simulink model "Data_Center_Module_Tier_1_No_Switching"  (R2024b)
settings: Solver=VariableStepAuto  StartTime=0.0  StopTime=60  RelTol=1e-3
undefined symbols (not defined in the file or in its folder): D1, Delta
libraries: spsThreePhaseSeriesRLCBranchLib x8, spsThreePhaseSeriesRLCLoadLib x7, spsThreePhaseProgrammableVoltageSourceLib x3, spsGroundLib x3, spsThreePhaseBreakerLib x3, spsThreePhaseTransformerTwoWindingsLib x2, spsPower3phInstantaneousLib x1, spsThreePhaseVIMeasurementLib x1, sps_lib x1
settings Model: Creator=Kapla  LastModifiedBy=Kapla

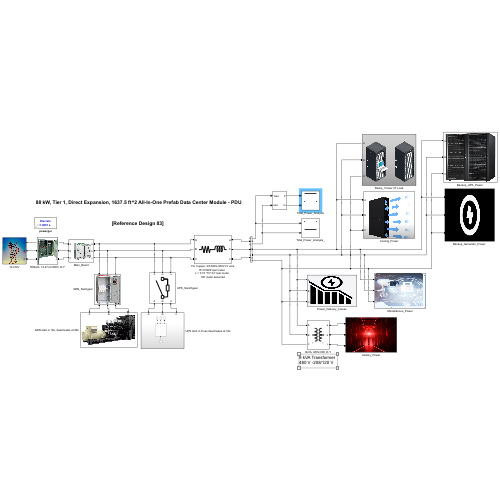
[thumbnail: Simulink's stored preview of the top-level diagram]
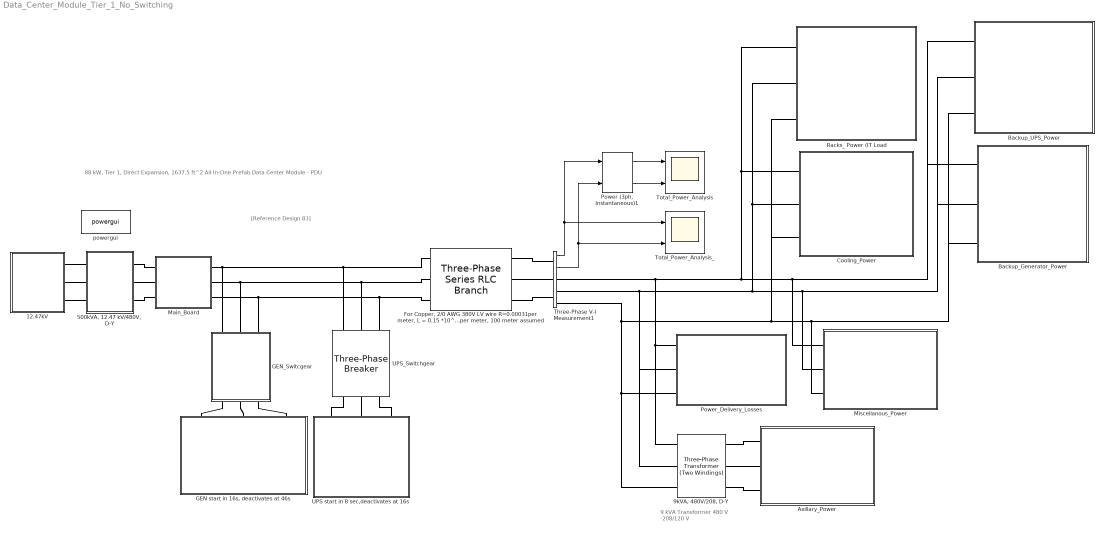
== system Data_Center_Module_Tier_1_No_Switching ==
  note: 9 kVA Transformer
      | 480 V -208/120 V
  note: [Reference Design 83]
  note: 88 kW, Tier 1, Direct Expansion, 1637.5 ft^2 All-In-One Prefab Data Center Module - PDU
  12.47kV : Subsystem
      mask Display: image('Power_Grid_.png');
  "500kVA, 12.47 kV/480V, D-Y" : Subsystem
      mask Display: image('Data_Center_Transformer_Tier_1.png');
  "9kVA, 480V/208, D-Y" : spsThreePhaseTransformerTwoWindingsLib/Three-Phase Transformer (Two Windings)  Winding1Connection=Y  Winding2Connection=Y  CoreType=Three single-phase transformers  SetSaturation=off  Hysteresis=off  DataFile='hysteresis'  SetInitialFlux=off  Measurements=None  UNITS=pu  NominalPower=[9e3 , 60 ]  Winding1=[ 480 , 0.002 , 0.08 ]  Winding2=[208 , 0.002 , 0.08 ]  Rm=500  Lm=500  L0=0.5  Saturation=[ 0,0 ; 0.0024,1.2 ; 1.0,1.52 ]  InitialFluxes=[ 0.8 , -0.8 , 0.7 ]  BreakLoop=off  DiscreteSolver=Trapezoidal iterative  DataType=off  TransfoNumber=1
  Axiliary_Power : Subsystem
      mask Display: image('Lighting_monitoring.png');
  "Backup_Generator_Power " : Subsystem
      mask Display: image('back up_generator_power.png');
  "Backup_UPS_Power " : Subsystem
      mask Display: image('UPS.png');
  Cooling_Power : Subsystem
      mask Display: image('Coolin.png');
  "For Copper, 2/0 AWG 380V LV wire R=0.00031per meter, L = 0.15 *10^-6 H per meter, 100 meter assumed " : spsThreePhaseSeriesRLCBranchLib/Three-Phase Series RLC Branch  LConnTagsString=A|B|C  RConnTagsString=A|B|C  BranchType=RL  Resistance=0.00031*100  Inductance=0.15e-6*100  Capacitance=[]  Measurements=None
  "GEN start in 16s, deactivates at 46s" : Subsystem
      mask Display: image('Back_up_Generator.png');
  GEN_Switcgear : Subsystem
      mask Display: image('GEN_Switch_gear_500kW.png');
  Main_Board : Subsystem
      mask Display: image('Main_Switch_Gear_Board.png');
  Miscellanous_Power : Subsystem
      mask Display: image('Data_Center_Security.png');
  "Power (3ph, Instantaneous)1" : spsPower3phInstantaneousLib/Power (3ph, Instantaneous)
  Power_Delivery_Losses : Subsystem
      mask Display: image('Power_Delivery_losses.png');
  Racks_ Power (IT Load : Subsystem
      mask Display: image('racks_server.png');
  Three-Phase V-I Measurement1 : spsThreePhaseVIMeasurementLib/Three-Phase V-I Measurement  VoltageMeasurement=phase-to-ground  SetLabelV=off  LabelV=V1  Vpu=off  VpuLL=off  CurrentMeasurement=yes  SetLabelI=off  LabelI=I1  Ipu=off  Pbase=100e6  Vbase=500e3  OutputType=Magnitude  PhasorSimulation=off  PSBequivalent=0
  Total_Power_Analysis : Scope  NumInputPorts=2
  Total_Power_Analysis_ : Scope  NumInputPorts=2
  UPS start in 8 sec,deactivates at 16s : Subsystem
  UPS_Switchgear : spsThreePhaseBreakerLib/Three-Phase Breaker  InitialState=open  SwitchA=on  SwitchB=on  SwitchC=on  SwitchTimes=[8 16]  External=off  BreakerResistance=0.01  SnubberResistance=1e6  SnubberCapacitance=inf  Measurements=None
  powergui : sps_lib/powergui  Priority=1  SimulationMode=Discrete  SampleTime=100e-6  frequency=60  Iterations=50  frequencyindice=60  Pbase=100e6  ErrMax=1e-4  UnitsV=kV  UnitsW=MW  buscounter=0  FunctionMessages=off  echomessages=off  EnableUseOfTLC=off  CurrentSourceSwitches=off  DisableSnubberDevices=off  DisableRonSwitches=off  DisableVfSwitches=off  DisplayEquations=off  AutomaticDiscreteSolvers=off  SolverType=Tustin/Backward Euler (TBE)  Interpol=off  ExternalGateDelay=off  methode=off  Ts=100  x0status=blocks  SPID=on  SwTol=0  HookPort=off  NonlinearTolerance=1e-4  nMaxIteration=100  ContinueOnMaxIteration=off  RestoreLinks=warning  ResistiveCurrentMeasurement=off  Frange=[0:2:500]  Ylog=off  Xlog=on  ShowGrid=off  save=off  variable=ZData  structure=0  ZoomFFT=off  StartTime=0.0  cycles=1  DisplayStyle=1  fundamental=60  FreqAxis=off  MaxFrequency=1000  frequencyindicesteady=1  RmsSteady=1  display=off
  wires:
  "Power (3ph, Instantaneous)1"/2 -> Total_Power_Analysis/2
  Three-Phase V-I Measurement1/1 -> "Power (3ph, Instantaneous)1"/1, Total_Power_Analysis_/1
  "Power (3ph, Instantaneous)1"/1 -> Total_Power_Analysis/1
  Three-Phase V-I Measurement1/2 -> "Power (3ph, Instantaneous)1"/2, Total_Power_Analysis_/2
  connections:
  Power_Delivery_Losses/LConn1 -- "9kVA, 480V/208, D-Y"/LConn1 -- "Backup_UPS_Power "/LConn1 -- "Backup_Generator_Power "/LConn1 -- Miscellanous_Power/LConn1 -- Racks_ Power (IT Load/LConn1 -- Cooling_Power/LConn1 -- Three-Phase V-I Measurement1/RConn1
  "For Copper, 2/0 AWG 380V LV wire R=0.00031per meter, L = 0.15 *10^-6 H per meter, 100 meter assumed "/RConn1 -- Three-Phase V-I Measurement1/LConn1
  "For Copper, 2/0 AWG 380V LV wire R=0.00031per meter, L = 0.15 *10^-6 H per meter, 100 meter assumed "/RConn3 -- Three-Phase V-I Measurement1/LConn3
  "9kVA, 480V/208, D-Y"/LConn2 -- Power_Delivery_Losses/LConn2 -- Three-Phase V-I Measurement1/RConn2 -- "Backup_UPS_Power "/LConn2 -- "Backup_Generator_Power "/LConn2 -- Miscellanous_Power/LConn2 -- Racks_ Power (IT Load/LConn2 -- Cooling_Power/LConn2
  Power_Delivery_Losses/LConn3 -- "9kVA, 480V/208, D-Y"/LConn3 -- "Backup_UPS_Power "/LConn3 -- "Backup_Generator_Power "/LConn3 -- Miscellanous_Power/LConn3 -- Racks_ Power (IT Load/LConn3 -- Cooling_Power/LConn3 -- Three-Phase V-I Measurement1/RConn3
  "For Copper, 2/0 AWG 380V LV wire R=0.00031per meter, L = 0.15 *10^-6 H per meter, 100 meter assumed "/RConn2 -- Three-Phase V-I Measurement1/LConn2
  Axiliary_Power/LConn1 -- "9kVA, 480V/208, D-Y"/RConn1
  Axiliary_Power/LConn3 -- "9kVA, 480V/208, D-Y"/RConn3
  Axiliary_Power/LConn2 -- "9kVA, 480V/208, D-Y"/RConn2
  UPS_Switchgear/LConn1 -- UPS start in 8 sec,deactivates at 16s/RConn1
  UPS_Switchgear/LConn2 -- UPS start in 8 sec,deactivates at 16s/RConn2
  UPS_Switchgear/LConn3 -- UPS start in 8 sec,deactivates at 16s/RConn3
  12.47kV/RConn1 -- "500kVA, 12.47 kV/480V, D-Y"/LConn1
  12.47kV/RConn2 -- "500kVA, 12.47 kV/480V, D-Y"/LConn2
  12.47kV/RConn3 -- "500kVA, 12.47 kV/480V, D-Y"/LConn3
  GEN_Switcgear/LConn1 -- "GEN start in 16s, deactivates at 46s"/RConn1
  GEN_Switcgear/LConn2 -- "GEN start in 16s, deactivates at 46s"/RConn2
  GEN_Switcgear/LConn3 -- "GEN start in 16s, deactivates at 46s"/RConn3
  "For Copper, 2/0 AWG 380V LV wire R=0.00031per meter, L = 0.15 *10^-6 H per meter, 100 meter assumed "/LConn3 -- Main_Board/RConn3 -- GEN_Switcgear/RConn3 -- UPS_Switchgear/RConn3
  GEN_Switcgear/RConn2 -- Main_Board/RConn2 -- UPS_Switchgear/RConn2 -- "For Copper, 2/0 AWG 380V LV wire R=0.00031per meter, L = 0.15 *10^-6 H per meter, 100 meter assumed "/LConn2
  GEN_Switcgear/RConn1 -- Main_Board/RConn1 -- UPS_Switchgear/RConn1 -- "For Copper, 2/0 AWG 380V LV wire R=0.00031per meter, L = 0.15 *10^-6 H per meter, 100 meter assumed "/LConn1
  Main_Board/LConn1 -- "500kVA, 12.47 kV/480V, D-Y"/RConn1
  "500kVA, 12.47 kV/480V, D-Y"/RConn2 -- Main_Board/LConn2
  Main_Board/LConn3 -- "500kVA, 12.47 kV/480V, D-Y"/RConn3

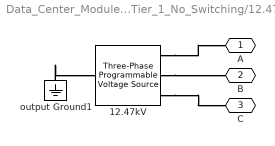
== system Data_Center_Module_Tier_1_No_Switching/12.47kV ==
  12.47kV : spsThreePhaseProgrammableVoltageSourceLib/Three-Phase Programmable Voltage Source  PositiveSequence="[12.4e3 0  60]"  VariationEntity=None  VariationType=Step  VariationTypeAlt=Step  VariationStep=-0.5  VariationRate=10  VariationMagnitude=0.5  VariationFrequency=1  VariationTiming=[0.2 1.2]  VariationPhaseA=off  Amplitudes=[1 0.8 1.2 1.0]  TimeValues=[0 0.1 0.15 0.2]  HarmonicGeneration=off  HarmonicA=[3 0.2 -25 0]  HarmonicB="[2 0.15  35 2]"  Timing="[0.05  3]"  BusType=swing  Pref=0  Qref=0  Qmin=-inf  Qmax=inf
  output Ground1 : spsGroundLib/Ground  LConnTagsString=a
  A : PMIOPort  Side=Right
  B : PMIOPort  Port=2  Side=Right
  C : PMIOPort  Port=3  Side=Right
  connections:
  output Ground1/LConn1 -- 12.47kV/LConn1
  12.47kV/RConn2 -- B/RConn1
  12.47kV/RConn3 -- C/RConn1
  12.47kV/RConn1 -- A/RConn1

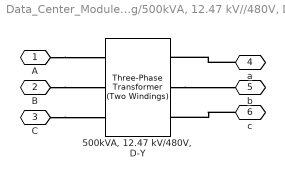
== system Data_Center_Module_Tier_1_No_Switching/500kVA, 12.47 kV//480V, D-Y ==
  "500kVA, 12.47 kV/480V, D-Y" : spsThreePhaseTransformerTwoWindingsLib/Three-Phase Transformer (Two Windings)  Winding1Connection=Delta (D1)  Winding2Connection=Y  CoreType=Three single-phase transformers  SetSaturation=off  Hysteresis=off  DataFile='hysteresis'  SetInitialFlux=off  Measurements=None  UNITS=pu  NominalPower=[ 500e3 , 60 ]  Winding1=[ 12.4e3 , 0.002 , 0.08 ]  Winding2=[ 0.48e3 , 0.002 , 0.08 ]  Rm=500  Lm=500  L0=0.5  Saturation=[ 0,0 ; 0.0024,1.2 ; 1.0,1.52 ]  InitialFluxes=[ 0.8 , -0.8 , 0.7 ]  BreakLoop=off  DiscreteSolver=Trapezoidal iterative  DataType=off  TransfoNumber=1
  A : PMIOPort  Side=Left
  B : PMIOPort  Port=2  Side=Left
  C : PMIOPort  Port=3  Side=Left
  a : PMIOPort  Port=4  Side=Right
  b : PMIOPort  Port=5  Side=Right
  c : PMIOPort  Port=6  Side=Right
  connections:
  "500kVA, 12.47 kV/480V, D-Y"/RConn2 -- b/RConn1
  A/RConn1 -- "500kVA, 12.47 kV/480V, D-Y"/LConn1
  a/RConn1 -- "500kVA, 12.47 kV/480V, D-Y"/RConn1
  B/RConn1 -- "500kVA, 12.47 kV/480V, D-Y"/LConn2
  c/RConn1 -- "500kVA, 12.47 kV/480V, D-Y"/RConn3
  C/RConn1 -- "500kVA, 12.47 kV/480V, D-Y"/LConn3

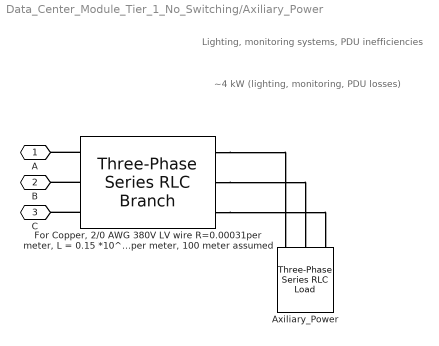
== system Data_Center_Module_Tier_1_No_Switching/Axiliary_Power ==
  note: ~4 kW (lighting, monitoring, PDU losses)
  note: Lighting, monitoring systems, PDU inefficiencies
  Axiliary_Power : spsThreePhaseSeriesRLCLoadLib/Three-Phase Series RLC Load  LConnTagsString=A|B|C  Configuration=Y (grounded)  NominalVoltage=208  Vabc=[1e3 1e3 1e3]  Vabcp=[1e3 1e3 1e3]  NominalFrequency=60  UnbalancedPower=off  ActivePower=4164  InductivePower=0  CapacitivePower=0  Pabc=[10e3 9e3 11e3]  QLabc=[100 90 110]  QCabc=[100 90 110]  Pabcp=[10e3 9e3 11e3]  QLabcp=[100 90 110]  QCabcp=[100 90 110]  Measurements=None  LoadType=constant Z
  "For Copper, 2/0 AWG 380V LV wire R=0.00031per meter, L = 0.15 *10^-6 H per meter, 100 meter assumed " : spsThreePhaseSeriesRLCBranchLib/Three-Phase Series RLC Branch  LConnTagsString=A|B|C  RConnTagsString=A|B|C  BranchType=RL  Resistance=0.00031*100  Inductance=0.15e-6*100  Capacitance=[]  Measurements=None
  A : PMIOPort  Side=Left
  B : PMIOPort  Port=2  Side=Left
  C : PMIOPort  Port=3  Side=Left
  connections:
  "For Copper, 2/0 AWG 380V LV wire R=0.00031per meter, L = 0.15 *10^-6 H per meter, 100 meter assumed "/LConn2 -- B/RConn1
  "For Copper, 2/0 AWG 380V LV wire R=0.00031per meter, L = 0.15 *10^-6 H per meter, 100 meter assumed "/LConn1 -- A/RConn1
  "For Copper, 2/0 AWG 380V LV wire R=0.00031per meter, L = 0.15 *10^-6 H per meter, 100 meter assumed "/LConn3 -- C/RConn1
  "For Copper, 2/0 AWG 380V LV wire R=0.00031per meter, L = 0.15 *10^-6 H per meter, 100 meter assumed "/RConn1 -- Axiliary_Power/LConn1
  "For Copper, 2/0 AWG 380V LV wire R=0.00031per meter, L = 0.15 *10^-6 H per meter, 100 meter assumed "/RConn2 -- Axiliary_Power/LConn2
  "For Copper, 2/0 AWG 380V LV wire R=0.00031per meter, L = 0.15 *10^-6 H per meter, 100 meter assumed "/RConn3 -- Axiliary_Power/LConn3

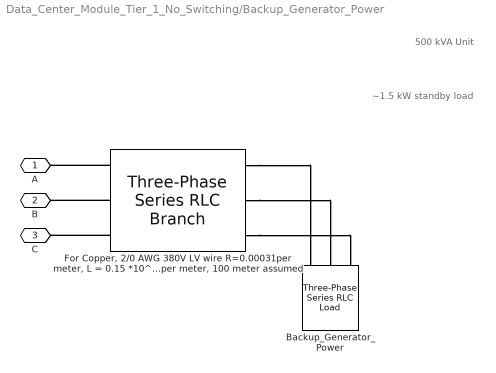
== system Data_Center_Module_Tier_1_No_Switching/Backup_Generator_Power  ==
  note: 500 kVA Unit
      |
      | ​
  note: ~1.5 kW standby load
      |
      | ​
  Backup_Generator_Power : spsThreePhaseSeriesRLCLoadLib/Three-Phase Series RLC Load  LConnTagsString=A|B|C  Configuration=Y (grounded)  NominalVoltage=480  Vabc=[1e3 1e3 1e3]  Vabcp=[1e3 1e3 1e3]  NominalFrequency=60  UnbalancedPower=off  ActivePower=11.81*1000  InductivePower=0  CapacitivePower=0  Pabc=[10e3 9e3 11e3]  QLabc=[100 90 110]  QCabc=[100 90 110]  Pabcp=[10e3 9e3 11e3]  QLabcp=[100 90 110]  QCabcp=[100 90 110]  Measurements=None  LoadType=constant Z
  "For Copper, 2/0 AWG 380V LV wire R=0.00031per meter, L = 0.15 *10^-6 H per meter, 100 meter assumed " : spsThreePhaseSeriesRLCBranchLib/Three-Phase Series RLC Branch  LConnTagsString=A|B|C  RConnTagsString=A|B|C  BranchType=RL  Resistance=0.00031*100  Inductance=0.15e-6*100  Capacitance=[]  Measurements=None
  A : PMIOPort  Side=Left
  B : PMIOPort  Port=2  Side=Left
  C : PMIOPort  Port=3  Side=Left
  connections:
  "For Copper, 2/0 AWG 380V LV wire R=0.00031per meter, L = 0.15 *10^-6 H per meter, 100 meter assumed "/LConn2 -- B/RConn1
  "For Copper, 2/0 AWG 380V LV wire R=0.00031per meter, L = 0.15 *10^-6 H per meter, 100 meter assumed "/LConn3 -- C/RConn1
  "For Copper, 2/0 AWG 380V LV wire R=0.00031per meter, L = 0.15 *10^-6 H per meter, 100 meter assumed "/LConn1 -- A/RConn1
  "For Copper, 2/0 AWG 380V LV wire R=0.00031per meter, L = 0.15 *10^-6 H per meter, 100 meter assumed "/RConn1 -- Backup_Generator_Power/LConn1
  "For Copper, 2/0 AWG 380V LV wire R=0.00031per meter, L = 0.15 *10^-6 H per meter, 100 meter assumed "/RConn2 -- Backup_Generator_Power/LConn2
  "For Copper, 2/0 AWG 380V LV wire R=0.00031per meter, L = 0.15 *10^-6 H per meter, 100 meter assumed "/RConn3 -- Backup_Generator_Power/LConn3

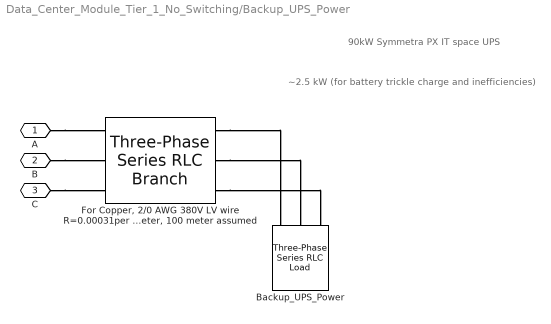
== system Data_Center_Module_Tier_1_No_Switching/Backup_UPS_Power  ==
  note: ~2.5 kW (for battery trickle charge and inefficiencies)
  note: 90kW Symmetra PX IT space UPS
      |
      | ​
  Backup_UPS_Power : spsThreePhaseSeriesRLCLoadLib/Three-Phase Series RLC Load  LConnTagsString=A|B|C  Configuration=Y (grounded)  NominalVoltage=480  Vabc=[1e3 1e3 1e3]  Vabcp=[1e3 1e3 1e3]  NominalFrequency=60  UnbalancedPower=off  ActivePower=2495  InductivePower=0  CapacitivePower=0  Pabc=[10e3 9e3 11e3]  QLabc=[100 90 110]  QCabc=[100 90 110]  Pabcp=[10e3 9e3 11e3]  QLabcp=[100 90 110]  QCabcp=[100 90 110]  Measurements=None  LoadType=constant Z
  "For Copper, 2/0 AWG 380V LV wire R=0.00031per meter, L = 0.15 *10^-6 H per meter, 100 meter assumed " : spsThreePhaseSeriesRLCBranchLib/Three-Phase Series RLC Branch  LConnTagsString=A|B|C  RConnTagsString=A|B|C  BranchType=RL  Resistance=0.00031*100  Inductance=0.15e-6*100  Capacitance=[]  Measurements=None
  A : PMIOPort  Side=Left
  B : PMIOPort  Port=2  Side=Left
  C : PMIOPort  Port=3  Side=Left
  connections:
  A/RConn1 -- "For Copper, 2/0 AWG 380V LV wire R=0.00031per meter, L = 0.15 *10^-6 H per meter, 100 meter assumed "/LConn1
  C/RConn1 -- "For Copper, 2/0 AWG 380V LV wire R=0.00031per meter, L = 0.15 *10^-6 H per meter, 100 meter assumed "/LConn3
  B/RConn1 -- "For Copper, 2/0 AWG 380V LV wire R=0.00031per meter, L = 0.15 *10^-6 H per meter, 100 meter assumed "/LConn2
  "For Copper, 2/0 AWG 380V LV wire R=0.00031per meter, L = 0.15 *10^-6 H per meter, 100 meter assumed "/RConn1 -- Backup_UPS_Power/LConn1
  "For Copper, 2/0 AWG 380V LV wire R=0.00031per meter, L = 0.15 *10^-6 H per meter, 100 meter assumed "/RConn2 -- Backup_UPS_Power/LConn2
  "For Copper, 2/0 AWG 380V LV wire R=0.00031per meter, L = 0.15 *10^-6 H per meter, 100 meter assumed "/RConn3 -- Backup_UPS_Power/LConn3

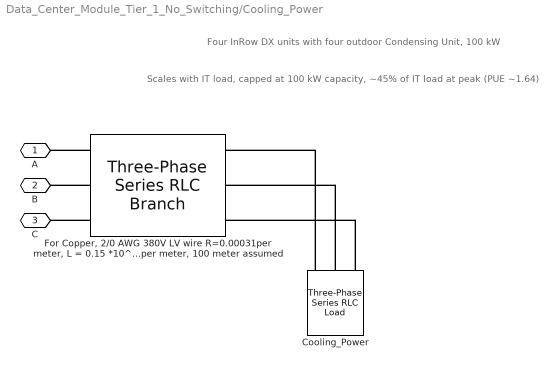
== system Data_Center_Module_Tier_1_No_Switching/Cooling_Power ==
  note: Four InRow DX units with four outdoor Condensing Unit, 100 kW
  note: Scales with IT load, capped at 100 kW capacity, ~45% of IT load at peak (PUE ~1.64)
  Cooling_Power : spsThreePhaseSeriesRLCLoadLib/Three-Phase Series RLC Load  LConnTagsString=A|B|C  Configuration=Y (grounded)  NominalVoltage=480  Vabc=[1e3 1e3 1e3]  Vabcp=[1e3 1e3 1e3]  NominalFrequency=60  UnbalancedPower=off  ActivePower=37326  InductivePower=37326*0.62  CapacitivePower=0  Pabc=[10e3 9e3 11e3]  QLabc=[100 90 110]  QCabc=[100 90 110]  Pabcp=[10e3 9e3 11e3]  QLabcp=[100 90 110]  QCabcp=[100 90 110]  Measurements=None  LoadType=constant Z
  "For Copper, 2/0 AWG 380V LV wire R=0.00031per meter, L = 0.15 *10^-6 H per meter, 100 meter assumed " : spsThreePhaseSeriesRLCBranchLib/Three-Phase Series RLC Branch  LConnTagsString=A|B|C  RConnTagsString=A|B|C  BranchType=RL  Resistance=0.00031*100  Inductance=0.15e-6*100  Capacitance=[]  Measurements=None
  A : PMIOPort  Side=Left
  B : PMIOPort  Port=2  Side=Left
  C : PMIOPort  Port=3  Side=Left
  connections:
  "For Copper, 2/0 AWG 380V LV wire R=0.00031per meter, L = 0.15 *10^-6 H per meter, 100 meter assumed "/LConn3 -- C/RConn1
  "For Copper, 2/0 AWG 380V LV wire R=0.00031per meter, L = 0.15 *10^-6 H per meter, 100 meter assumed "/LConn2 -- B/RConn1
  "For Copper, 2/0 AWG 380V LV wire R=0.00031per meter, L = 0.15 *10^-6 H per meter, 100 meter assumed "/LConn1 -- A/RConn1
  Cooling_Power/LConn1 -- "For Copper, 2/0 AWG 380V LV wire R=0.00031per meter, L = 0.15 *10^-6 H per meter, 100 meter assumed "/RConn1
  Cooling_Power/LConn2 -- "For Copper, 2/0 AWG 380V LV wire R=0.00031per meter, L = 0.15 *10^-6 H per meter, 100 meter assumed "/RConn2
  Cooling_Power/LConn3 -- "For Copper, 2/0 AWG 380V LV wire R=0.00031per meter, L = 0.15 *10^-6 H per meter, 100 meter assumed "/RConn3

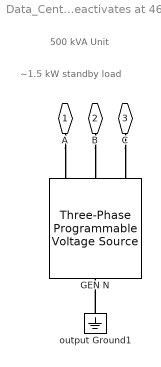
== system Data_Center_Module_Tier_1_No_Switching/GEN start in 16s, deactivates at 46s ==
  note: ~1.5 kW standby load
      |
      | ​
  note: 500 kVA Unit
      |
      | ​
  GEN N : spsThreePhaseProgrammableVoltageSourceLib/Three-Phase Programmable Voltage Source  PositiveSequence="[480 0  60]"  VariationEntity=None  VariationType=Step  VariationTypeAlt=Step  VariationStep=-0.5  VariationRate=10  VariationMagnitude=0.5  VariationFrequency=1  VariationTiming=[0.2 1.2]  VariationPhaseA=off  Amplitudes=[1 0.8 1.2 1.0]  TimeValues=[0 0.1 0.15 0.2]  HarmonicGeneration=off  HarmonicA=[3 0.2 -25 0]  HarmonicB="[2 0.15  35 2]"  Timing="[0.05  3]"  BusType=PV  Pref=500e3  Qref=0  Qmin=-inf  Qmax=inf
  output Ground1 : spsGroundLib/Ground  LConnTagsString=a
  A : PMIOPort  Side=Right
  B : PMIOPort  Port=2  Side=Right
  C : PMIOPort  Port=3  Side=Right
  connections:
  C/RConn1 -- GEN N/RConn3
  A/RConn1 -- GEN N/RConn1
  B/RConn1 -- GEN N/RConn2
  output Ground1/LConn1 -- GEN N/LConn1

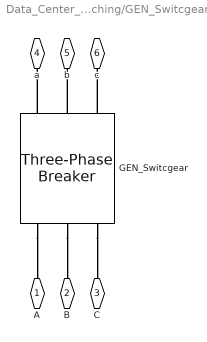
== system Data_Center_Module_Tier_1_No_Switching/GEN_Switcgear ==
  GEN_Switcgear : spsThreePhaseBreakerLib/Three-Phase Breaker  InitialState=open  SwitchA=on  SwitchB=on  SwitchC=on  SwitchTimes=[16 46]  External=off  BreakerResistance=0.01  SnubberResistance=1e6  SnubberCapacitance=inf  Measurements=None
  A : PMIOPort  Side=Left
  B : PMIOPort  Port=2  Side=Left
  C : PMIOPort  Port=3  Side=Left
  a : PMIOPort  Port=4  Side=Right
  b : PMIOPort  Port=5  Side=Right
  c : PMIOPort  Port=6  Side=Right
  connections:
  GEN_Switcgear/RConn2 -- b/RConn1
  GEN_Switcgear/RConn1 -- a/RConn1
  GEN_Switcgear/LConn1 -- A/RConn1
  GEN_Switcgear/LConn3 -- C/RConn1
  GEN_Switcgear/RConn3 -- c/RConn1
  GEN_Switcgear/LConn2 -- B/RConn1

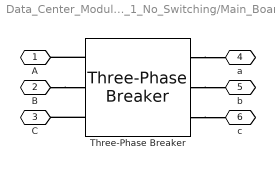
== system Data_Center_Module_Tier_1_No_Switching/Main_Board ==
  Three-Phase Breaker : spsThreePhaseBreakerLib/Three-Phase Breaker  InitialState=closed  SwitchA=on  SwitchB=on  SwitchC=on  SwitchTimes=[8 46]  External=off  BreakerResistance=0.01  SnubberResistance=1e6  SnubberCapacitance=inf  Measurements=None
  A : PMIOPort  Side=Left
  B : PMIOPort  Port=2  Side=Left
  C : PMIOPort  Port=3  Side=Left
  a : PMIOPort  Port=4  Side=Right
  b : PMIOPort  Port=5  Side=Right
  c : PMIOPort  Port=6  Side=Right
  connections:
  Three-Phase Breaker/RConn1 -- a/RConn1
  Three-Phase Breaker/RConn3 -- c/RConn1
  Three-Phase Breaker/LConn3 -- C/RConn1
  B/RConn1 -- Three-Phase Breaker/LConn2
  Three-Phase Breaker/RConn2 -- b/RConn1
  Three-Phase Breaker/LConn1 -- A/RConn1

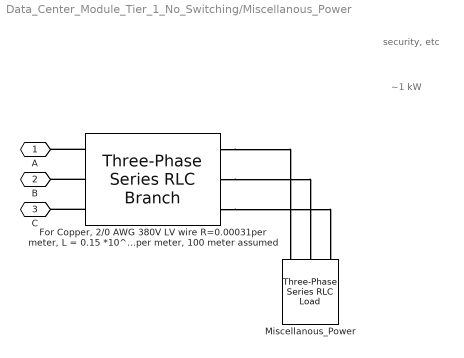
== system Data_Center_Module_Tier_1_No_Switching/Miscellanous_Power ==
  note: security, etc
      |
      | ​
      |
      | ​
  note: ~1 kW
  "For Copper, 2/0 AWG 380V LV wire R=0.00031per meter, L = 0.15 *10^-6 H per meter, 100 meter assumed " : spsThreePhaseSeriesRLCBranchLib/Three-Phase Series RLC Branch  LConnTagsString=A|B|C  RConnTagsString=A|B|C  BranchType=RL  Resistance=0.00031*100  Inductance=0.15e-6*100  Capacitance=[]  Measurements=None
  Miscellanous_Power : spsThreePhaseSeriesRLCLoadLib/Three-Phase Series RLC Load  LConnTagsString=A|B|C  Configuration=Y (grounded)  NominalVoltage=480  Vabc=[1e3 1e3 1e3]  Vabcp=[1e3 1e3 1e3]  NominalFrequency=60  UnbalancedPower=off  ActivePower=1131  InductivePower=0  CapacitivePower=0  Pabc=[10e3 9e3 11e3]  QLabc=[100 90 110]  QCabc=[100 90 110]  Pabcp=[10e3 9e3 11e3]  QLabcp=[100 90 110]  QCabcp=[100 90 110]  Measurements=None  LoadType=constant Z
  A : PMIOPort  Side=Left
  B : PMIOPort  Port=2  Side=Left
  C : PMIOPort  Port=3  Side=Left
  connections:
  "For Copper, 2/0 AWG 380V LV wire R=0.00031per meter, L = 0.15 *10^-6 H per meter, 100 meter assumed "/LConn2 -- B/RConn1
  "For Copper, 2/0 AWG 380V LV wire R=0.00031per meter, L = 0.15 *10^-6 H per meter, 100 meter assumed "/LConn1 -- A/RConn1
  "For Copper, 2/0 AWG 380V LV wire R=0.00031per meter, L = 0.15 *10^-6 H per meter, 100 meter assumed "/LConn3 -- C/RConn1
  "For Copper, 2/0 AWG 380V LV wire R=0.00031per meter, L = 0.15 *10^-6 H per meter, 100 meter assumed "/RConn1 -- Miscellanous_Power/LConn1
  "For Copper, 2/0 AWG 380V LV wire R=0.00031per meter, L = 0.15 *10^-6 H per meter, 100 meter assumed "/RConn2 -- Miscellanous_Power/LConn2
  "For Copper, 2/0 AWG 380V LV wire R=0.00031per meter, L = 0.15 *10^-6 H per meter, 100 meter assumed "/RConn3 -- Miscellanous_Power/LConn3

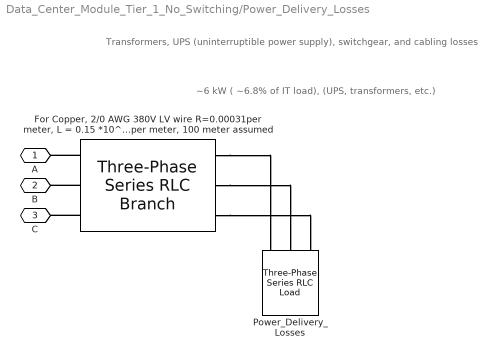
== system Data_Center_Module_Tier_1_No_Switching/Power_Delivery_Losses ==
  note: ~6 kW ( ~6.8% of IT load), (UPS, transformers, etc.)
  note: Transformers, UPS (uninterruptible power supply), switchgear, and cabling losses
  "For Copper, 2/0 AWG 380V LV wire R=0.00031per meter, L = 0.15 *10^-6 H per meter, 100 meter assumed " : spsThreePhaseSeriesRLCBranchLib/Three-Phase Series RLC Branch  LConnTagsString=A|B|C  RConnTagsString=A|B|C  BranchType=RL  Resistance=0.00031*100  Inductance=0.15e-6*100  Capacitance=[]  Measurements=None
  Power_Delivery_Losses : spsThreePhaseSeriesRLCLoadLib/Three-Phase Series RLC Load  LConnTagsString=A|B|C  Configuration=Y (grounded)  NominalVoltage=480  Vabc=[1e3 1e3 1e3]  Vabcp=[1e3 1e3 1e3]  NominalFrequency=60  UnbalancedPower=off  ActivePower=5309  InductivePower=0  CapacitivePower=0  Pabc=[10e3 9e3 11e3]  QLabc=[100 90 110]  QCabc=[100 90 110]  Pabcp=[10e3 9e3 11e3]  QLabcp=[100 90 110]  QCabcp=[100 90 110]  Measurements=None  LoadType=constant Z
  A : PMIOPort  Side=Left
  B : PMIOPort  Port=2  Side=Left
  C : PMIOPort  Port=3  Side=Left
  connections:
  "For Copper, 2/0 AWG 380V LV wire R=0.00031per meter, L = 0.15 *10^-6 H per meter, 100 meter assumed "/LConn3 -- C/RConn1
  "For Copper, 2/0 AWG 380V LV wire R=0.00031per meter, L = 0.15 *10^-6 H per meter, 100 meter assumed "/LConn1 -- A/RConn1
  "For Copper, 2/0 AWG 380V LV wire R=0.00031per meter, L = 0.15 *10^-6 H per meter, 100 meter assumed "/LConn2 -- B/RConn1
  "For Copper, 2/0 AWG 380V LV wire R=0.00031per meter, L = 0.15 *10^-6 H per meter, 100 meter assumed "/RConn1 -- Power_Delivery_Losses/LConn1
  "For Copper, 2/0 AWG 380V LV wire R=0.00031per meter, L = 0.15 *10^-6 H per meter, 100 meter assumed "/RConn2 -- Power_Delivery_Losses/LConn2
  "For Copper, 2/0 AWG 380V LV wire R=0.00031per meter, L = 0.15 *10^-6 H per meter, 100 meter assumed "/RConn3 -- Power_Delivery_Losses/LConn3

== system Data_Center_Module_Tier_1_No_Switching/Racks_ Power (IT Load ==
  note: Servers, storage, networking equipment. 88 kW, 11 racks and 8 kW/rack
  note: 88 kW max,11 racks, 8 kW per rack, varies with workload (50% idle, 100% peak)
  "For Copper, 2/0 AWG 380V LV wire R=0.00031per meter, L = 0.15 *10^-6 H per meter, 100 meter assumed " : spsThreePhaseSeriesRLCBranchLib/Three-Phase Series RLC Branch  LConnTagsString=A|B|C  RConnTagsString=A|B|C  BranchType=RL  Resistance=0.00031*100  Inductance=0.15e-6*100  Capacitance=[]  Measurements=None
  Racks_ Power (IT Load : spsThreePhaseSeriesRLCLoadLib/Three-Phase Series RLC Load  LConnTagsString=A|B|C  Configuration=Y (grounded)  NominalVoltage=480  Vabc=[1e3 1e3 1e3]  Vabcp=[1e3 1e3 1e3]  NominalFrequency=60  UnbalancedPower=off  ActivePower=86875  InductivePower=86875*0.33  CapacitivePower=0  Pabc=[10e3 9e3 11e3]  QLabc=[100 90 110]  QCabc=[100 90 110]  Pabcp=[10e3 9e3 11e3]  QLabcp=[100 90 110]  QCabcp=[100 90 110]  Measurements=None  LoadType=constant Z
  A : PMIOPort  Side=Left
  B : PMIOPort  Port=2  Side=Left
  C : PMIOPort  Port=3  Side=Left
  connections:
  C/RConn1 -- "For Copper, 2/0 AWG 380V LV wire R=0.00031per meter, L = 0.15 *10^-6 H per meter, 100 meter assumed "/LConn3
  B/RConn1 -- "For Copper, 2/0 AWG 380V LV wire R=0.00031per meter, L = 0.15 *10^-6 H per meter, 100 meter assumed "/LConn2
  A/RConn1 -- "For Copper, 2/0 AWG 380V LV wire R=0.00031per meter, L = 0.15 *10^-6 H per meter, 100 meter assumed "/LConn1
  "For Copper, 2/0 AWG 380V LV wire R=0.00031per meter, L = 0.15 *10^-6 H per meter, 100 meter assumed "/RConn1 -- Racks_ Power (IT Load/LConn1
  "For Copper, 2/0 AWG 380V LV wire R=0.00031per meter, L = 0.15 *10^-6 H per meter, 100 meter assumed "/RConn2 -- Racks_ Power (IT Load/LConn2
  "For Copper, 2/0 AWG 380V LV wire R=0.00031per meter, L = 0.15 *10^-6 H per meter, 100 meter assumed "/RConn3 -- Racks_ Power (IT Load/LConn3

== system Data_Center_Module_Tier_1_No_Switching/UPS start in 8 sec,deactivates at 16s ==
  UPS : spsThreePhaseProgrammableVoltageSourceLib/Three-Phase Programmable Voltage Source  PositiveSequence="[480 0  60]"  VariationEntity=None  VariationType=Step  VariationTypeAlt=Step  VariationStep=-0.5  VariationRate=10  VariationMagnitude=0.5  VariationFrequency=1  VariationTiming=[0.2 1.2]  VariationPhaseA=off  Amplitudes=[1 0.8 1.2 1.0]  TimeValues=[0 0.1 0.15 0.2]  HarmonicGeneration=off  HarmonicA=[3 0.2 -25 0]  HarmonicB="[2 0.15  35 2]"  Timing="[0.05  3]"  BusType=swing  Pref=500e3  Qref=0  Qmin=-inf  Qmax=inf
  output Ground1 : spsGroundLib/Ground  LConnTagsString=a
  A : PMIOPort  Side=Right
  B : PMIOPort  Port=2  Side=Right
  C : PMIOPort  Port=3  Side=Right
  connections:
  UPS/RConn2 -- B/RConn1
  UPS/RConn1 -- A/RConn1
  UPS/RConn3 -- C/RConn1
  output Ground1/LConn1 -- UPS/LConn1
